simulink model "disturbed_subsystem_old"  (Simulink 9.0)
settings: Solver=ode5  StartTime=0.0  StopTime=30  RelTol=1e-3  AbsTol=1e-6
model workspace: external: MATLAB File workspace.m (data not in the file)
values from neighbouring files (symbols this model uses):
  DOWN_TABLE = [0 5 20 35 ... (first row only)    [workspace.m]
  DOWN_TH_BP = [0; 5; 40; 50; 90; 100]    [workspace.m]
  EMAP = [-40 -44 -49 -53 -57 -61 -65 -70 -74 -78 -82 ... (first row only)    [workspace.m]
  Iei = 0.021991488283555904    (= 0.0219914882836)    [workspace.m]
  NE_VEC = [799.99999999999989 1200 1599.9999999999998 1999.9999999999998            2400 2800.0000000000005 3199.9999999999995 3599.9999999999995            3999.9999999999995 4400 4800]    [workspace.m]
  TH_VEC = [0; 20; 30; 40; 50; 60; 70; 80; 90; 100]    [workspace.m]
  UP_TABLE = [12 30 50 1.0E+6 ... (first row only)    [workspace.m]
  UP_TH_BP = [0; 25; 35; 50; 90; 100]    [workspace.m]
undefined symbols (not defined in the file): CONVERTER_DATA, VEHICLE_DATA
Description:
  | Modeling an Automatic Transmission Controller
  | 
  | In this example, Simulink(R) is used to model an automotive drivetrain. Stateflow(R)
  | enhances the Simulink model with its representation of the transmission
  | control logic. Simulink provides a powerful environment for the modeling and
  | simulation of dynamic systems and processes. In many systems, though,
  | supervisory functions like changing modes or invoking new gain schedules must
  | respond to events that may occur and conditions that develop over time. As a
  | result, the environment requires a language capable of managing these multiple
  | modes and developing conditions. In the following example, Stateflow
  | demonstrates its strength in this capacity by performing the function of gear
  | selection in an automatic transmission. This function is combined with the
  | drivetrain dynamics in a natural and intuitive manner by incorporating a
  | Stateflow block in the Simulink block diagram.
settings Model: SuppressorTable=22 serialization::archive 11 0 6 0 0 0 1 0  DataTypeOverride=Double  MinMaxOverflowLogging=ForceOff  FPTRunName=Active  Creator=The MathWorks, Inc.  LastModifiedBy=luigi  ExtModeTrigMode=oneshot  ExtModeArmWhenConnect=off  ExtModeAutoUpdateStatusClock=off
settings DataIOCC: SaveFormat=StructureWithTime  SaveOutput=off  SaveTime=off  SignalLoggingName=sldemo_autotrans_output
settings OptimizationCC: BlockReduction=off  ExpressionDepthLimit=2147483647  InitFltsAndDblsToZero=on
settings DebuggingCC: SignalInfNanChecking=error  SaveWithParameterizedLinksMsg=none  UnderspecifiedInitializationDetection=Simplified  MergeDetectMultiDrivingBlocksExec=error  CheckExecutionContextPreStartOutputMsg=on  CheckExecutionContextRuntimeOutputMsg=on  MultiTaskCondExecSysMsg=none  SigSpecEnsureSampleTimeMsg=none  IntegerOverflowMsg=none  FcnCallInpInsideContextMsg=warning  SignalLabelMismatchMsg=error  UnconnectedInputMsg=error  UnconnectedOutputMsg=error  UnconnectedLineMsg=error  UniqueDataStoreMsg=error  BusObjectLabelMismatch=error  RootOutportRequireBusObject=error  StateNameClashWarn=warning  StrictBusMsg=ErrorOnBusTreatedAsVector  NonBusSignalsTreatedAsBus=error  IntegerSaturationMsg=none
settings HardwareCC: ProdIntDivRoundTo=Floor
settings SFSimCC: SFSimEcho=off  SimParseCustomCode=off
settings GRTTargetCC: TargetFcnLib=ansi_tfl_tmw.mat  GeneratePreprocessorConditionals=Disable all  CombineOutputUpdateFcns=off  GRTInterface=on
settings ConfigComp: CovMetricSettings=dcmtr  CovHTMLOptions=-aTS=1 -bRG=1 -bTC=1 -hTR=0 -nFC=0 -scm=1 -bcm=1 -xEv=0  CovHtmlReporting=off

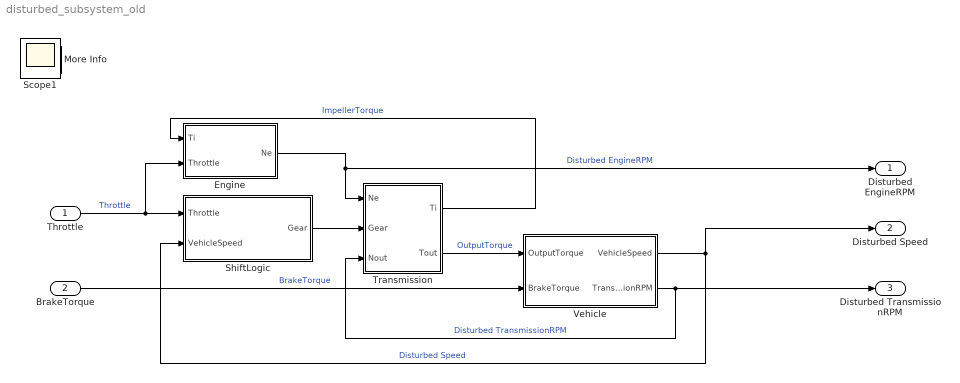
== system disturbed_subsystem_old ==
  Throttle : Inport
  BrakeTorque : Inport  Port=2
  Engine : Subsystem
  More Info : Subsystem
      settings: OpenFcn=showdemo(bdroot(gcb))
      mask Display: disp('?')
  ShiftLogic : Stateflow chart  TreatAsAtomicUnit=on
  Transmission : Subsystem
  Vehicle : Subsystem  mask(vehicle model){Rfd=VEHICLE_DATA(1), rload0=VEHICLE_DATA(2), rload2=VEHICLE_DATA(3), Rw=VEHICLE_DATA(4), Iv=VEHICLE_DATA(5), N20=VEHICLE_DATA(6)/VEHICLE_DATA(4)*VEHICLE_DATA(1)}
      mask prompts: Rfd "final drive ratio"; rload0 "drag friction at wheels"; rload2 "aerodynamic drag"; Rw "wheel radius"; Iv "vehicle inertia"; N20 "initial transmission output speed"
      mask help: vehicle dynamics: torque input from trans., outputs are input speed (transmission output) and vehicle speed
      mask Display: image([matlabroot,'/toolbox/simulink/simdemos/automotive/html/NSX_3Colors.jpg'])
  Disturbed EngineRPM : Outport
  Disturbed Speed : Outport  Port=2
  Disturbed TransmissionRPM : Outport  Port=3
  Scope1 : Scope
  wires:
  Transmission/1(Ti) -> Engine/1(Ti)  "ImpellerTorque"
  Engine/1(Ne) -> Disturbed EngineRPM/1, Transmission/1(Ne)  "Disturbed EngineRPM"
  Transmission/2(Tout) -> Vehicle/1(OutputTorque)  "OutputTorque"
  Vehicle/2(TransmissionRPM) -> Transmission/3(Nout), Disturbed TransmissionRPM/1  "Disturbed TransmissionRPM"
  ShiftLogic/1(Gear) -> Transmission/2(Gear)
  Vehicle/1(VehicleSpeed) -> Disturbed Speed/1, ShiftLogic/2(VehicleSpeed)  "Disturbed Speed"
  Throttle/1 -> Engine/2(Throttle), ShiftLogic/1(Throttle)  "Throttle"
  BrakeTorque/1 -> Vehicle/2(BrakeTorque)  "BrakeTorque"

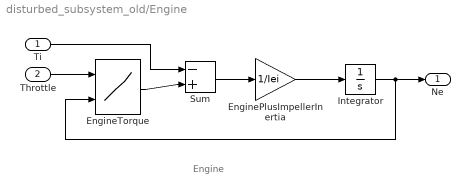
== system disturbed_subsystem_old/Engine ==
  note: Engine
  Ti : Inport  Unit=ft*lbf@torque
  Throttle : Inport  Port=2  Unit=%
  EnginePlusImpellerInertia : Gain  Gain=1/Iei  SaturateOnIntegerOverflow=on  OutDataTypeStr=Inherit: Same as input  ParamDataTypeStr=Inherit: Same as input
  EngineTorque : Lookup_n-D  BreakpointsForDimension1=TH_VEC  BreakpointsForDimension2=NE_VEC  Table=EMAP  InputSameDT=on
  Integrator : Integrator  InitialCondition=1000  LimitOutput=on  UpperSaturationLimit=6000  LowerSaturationLimit=600  ZeroCross=off
  Sum : Sum  Inputs=-+  SaturateOnIntegerOverflow=on  InputSameDT=on  OutDataTypeStr=Inherit: Same as first input
  Ne : Outport  Unit=rpm
  wires:
  Ti/1 -> Sum/1
  Throttle/1 -> EngineTorque/1
  Integrator/1 -> EngineTorque/2, Ne/1
  Sum/1 -> EnginePlusImpellerInertia/1
  EnginePlusImpellerInertia/1 -> Integrator/1
  EngineTorque/1 -> Sum/2

== system disturbed_subsystem_old/More Info ==

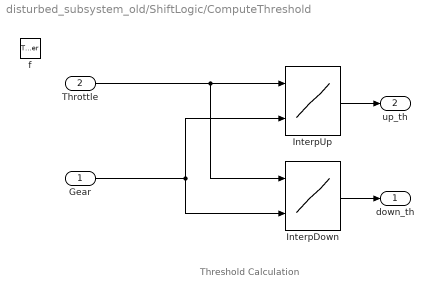
== system disturbed_subsystem_old/ShiftLogic/ComputeThreshold ==
  note: Threshold Calculation
  Gear : Inport
  Throttle : Inport  Port=2
  f : TriggerPort  TriggerType=function-call  VariantControl=(inherit)
      settings: CopyFcn=Stateflow.SLINSF.SimulinkMan.removeBlockPreDeleteFcn  PreDeleteFcn=Stateflow.SLINSF.SimulinkMan.unsafePredeleteFcn
  InterpDown : Lookup_n-D  BreakpointsForDimension1=DOWN_TH_BP  BreakpointsForDimension2=[1:4]  Table=DOWN_TABLE  OutDataTypeStr=double  LockScale=on
  InterpUp : Lookup_n-D  BreakpointsForDimension1=UP_TH_BP  BreakpointsForDimension2=[1:4]  Table=UP_TABLE  OutDataTypeStr=double  LockScale=on
  down_th : Outport  InitialOutput=0
  up_th : Outport  Port=2  InitialOutput=0
  wires:
  InterpUp/1 -> up_th/1
  InterpDown/1 -> down_th/1
  Throttle/1 -> InterpDown/1, InterpUp/1
  Gear/1 -> InterpDown/2, InterpUp/2

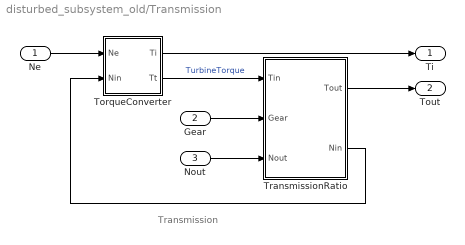
== system disturbed_subsystem_old/Transmission ==
  note: Transmission
  Ne : Inport  Unit=rpm
  Gear : Inport  Port=2  Unit=1
  Nout : Inport  Port=3  Unit=rpm
  TorqueConverter : Subsystem  mask(torque converter){speedratio=CONVERTER_DATA(:,1), Kfactor=CONVERTER_DATA(:,2), Torkratio=CONVERTER_DATA(:,3)}
      mask prompts: speedratio "speed ratio"; Kfactor "K factor"; Torkratio "torque ratio"
      mask help: torque converter
      mask Help: Torque converter input and output torques are computed as a function of the input and output speeds
      mask Display: plot([cos([90:10:450]*pi/180),.63*cos([90:10:450]*pi/180),.63*cos([90:10:240]*pi/180),cos([240:10:300]*pi/180),.63*cos([300]*pi/180)],[sin([90:10:450]*pi/180),.63*sin([90:10:450]*pi/180)+.1,.63*sin([90:10:240]*pi/180)+.1,sin([240:10:300]*pi/180),.63*sin([300]*pi/180)+.1])
  TransmissionRatio : Subsystem
  Ti : Outport  Unit=ft*lbf@torque
  Tout : Outport  Port=2  Unit=ft*lbf@torque
  wires:
  TransmissionRatio/1(Tout) -> Tout/1
  TorqueConverter/1(Ti) -> Ti/1
  Nout/1 -> TransmissionRatio/3(Nout)
  Gear/1 -> TransmissionRatio/2(Gear)
  Ne/1 -> TorqueConverter/1(Ne)
  TransmissionRatio/2(Nin) -> TorqueConverter/2(Nin)
  TorqueConverter/2(Tt) -> TransmissionRatio/1(Tin)  "TurbineTorque"

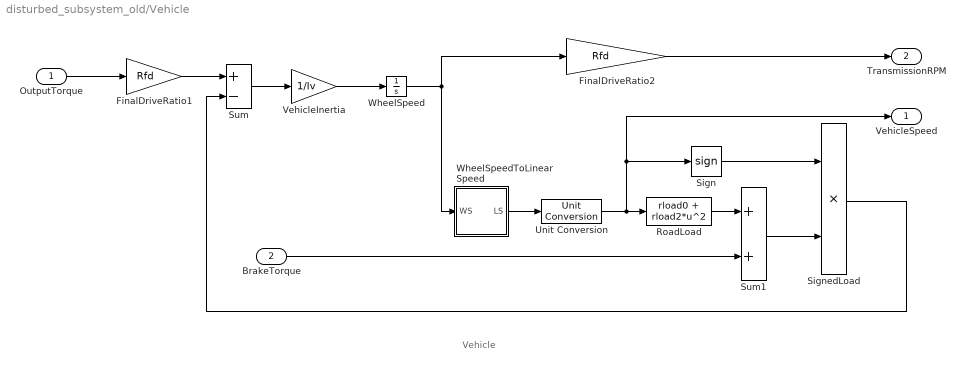
== system disturbed_subsystem_old/Vehicle ==
  note: Vehicle
  OutputTorque : Inport  Unit=ft*lbf@torque
  BrakeTorque : Inport  Port=2  Unit=ft*lbf@torque
  FinalDriveRatio1 : Gain  Gain=Rfd  SaturateOnIntegerOverflow=on  OutDataTypeStr=Inherit: Same as input  ParamDataTypeStr=Inherit: Same as input
  FinalDriveRatio2 : Gain  Gain=Rfd  SaturateOnIntegerOverflow=on  OutDataTypeStr=Inherit: Same as input  ParamDataTypeStr=Inherit: Same as input
  RoadLoad : Fcn  Expr=rload0 + rload2*u^2
  Sign : Signum
  SignedLoad : Product  SaturateOnIntegerOverflow=on  InputSameDT=on  OutDataTypeStr=Inherit: Same as first input
  Sum : Sum  Inputs=+-  SaturateOnIntegerOverflow=on  InputSameDT=on  OutDataTypeStr=Inherit: Same as first input
  Sum1 : Sum  SaturateOnIntegerOverflow=on  InputSameDT=on  OutDataTypeStr=Inherit: Same as first input
  Unit Conversion : UnitConversion
  VehicleInertia : Gain  Gain=1/Iv  SaturateOnIntegerOverflow=on  OutDataTypeStr=Inherit: Same as input  ParamDataTypeStr=Inherit: Same as input
  WheelSpeed : Integrator  InitialCondition=N20/Rfd  ZeroCross=off
  WheelSpeedToLinearSpeed : Subsystem
  VehicleSpeed : Outport  Unit=mph
  TransmissionRPM : Outport  Port=2  Unit=rpm
  wires:
  FinalDriveRatio2/1 -> TransmissionRPM/1
  BrakeTorque/1 -> Sum1/2
  Sum1/1 -> SignedLoad/2
  RoadLoad/1 -> Sum1/1
  Sign/1 -> SignedLoad/1
  SignedLoad/1 -> Sum/2
  OutputTorque/1 -> FinalDriveRatio1/1
  VehicleInertia/1 -> WheelSpeed/1
  Sum/1 -> VehicleInertia/1
  Unit Conversion/1 -> VehicleSpeed/1, Sign/1, RoadLoad/1
  WheelSpeed/1 -> WheelSpeedToLinearSpeed/1(WS), FinalDriveRatio2/1
  FinalDriveRatio1/1 -> Sum/1
  WheelSpeedToLinearSpeed/1(LS) -> Unit Conversion/1

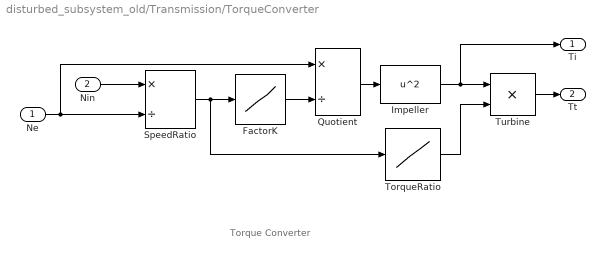
== system disturbed_subsystem_old/Transmission/TorqueConverter ==
  note: Torque Converter
  Ne : Inport
  Nin : Inport  Port=2
  FactorK : Lookup_n-D  NumberOfTableDimensions=1  BreakpointsForDimension1=speedratio  Table=Kfactor  SaturateOnIntegerOverflow=on  InputSameDT=on
  Impeller : Fcn  Expr=u^2
  Quotient : Product  Inputs=*/  SaturateOnIntegerOverflow=on  InputSameDT=on  OutDataTypeStr=Inherit: Same as first input
  SpeedRatio : Product  Inputs=*/  SaturateOnIntegerOverflow=on  InputSameDT=on  OutDataTypeStr=Inherit: Same as first input
  TorqueRatio : Lookup_n-D  NumberOfTableDimensions=1  BreakpointsForDimension1=speedratio  Table=Torkratio  SaturateOnIntegerOverflow=on  InputSameDT=on
  Turbine : Product  SaturateOnIntegerOverflow=on  InputSameDT=on  OutDataTypeStr=Inherit: Same as first input
  Ti : Outport
  Tt : Outport  Port=2
  wires:
  TorqueRatio/1 -> Turbine/2
  Quotient/1 -> Impeller/1
  FactorK/1 -> Quotient/2
  SpeedRatio/1 -> TorqueRatio/1, FactorK/1
  Impeller/1 -> Turbine/1, Ti/1
  Turbine/1 -> Tt/1
  Ne/1 -> SpeedRatio/2, Quotient/1
  Nin/1 -> SpeedRatio/1

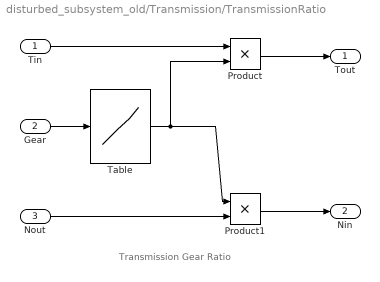
== system disturbed_subsystem_old/Transmission/TransmissionRatio ==
  note: Transmission Gear Ratio
  Tin : Inport  Unit=ft*lbf@torque
  Gear : Inport  Port=2  Unit=1
  Nout : Inport  Port=3  Unit=rpm
  Product : Product  SaturateOnIntegerOverflow=on  InputSameDT=on  OutDataTypeStr=Inherit: Same as first input
  Product1 : Product  SaturateOnIntegerOverflow=on  InputSameDT=on  OutDataTypeStr=Inherit: Same as first input
  Table : Lookup_n-D  NumberOfTableDimensions=1  BreakpointsForDimension1=[1 2 3 4]  Table=[2.393 1.450 1.000 0.677]  OutDataTypeStr=double  SaturateOnIntegerOverflow=on  InputSameDT=on  LockScale=on
  Tout : Outport  Unit=ft*lbf@torque
  Nin : Outport  Port=2  Unit=rpm
  wires:
  Table/1 -> Product1/1, Product/2
  Nout/1 -> Product1/2
  Product1/1 -> Nin/1
  Product/1 -> Tout/1
  Tin/1 -> Product/1
  Gear/1 -> Table/1

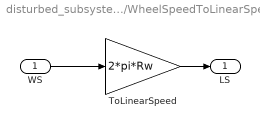
== system disturbed_subsystem_old/Vehicle/WheelSpeedToLinearSpeed ==
  WS : Inport  Unit=rpm
  ToLinearSpeed : Gain  Gain=2*pi*Rw  SaturateOnIntegerOverflow=on  OutDataTypeStr=Inherit: Same as input  ParamDataTypeStr=Inherit: Same as input
  LS : Outport  Unit=ft/min
  wires:
  ToLinearSpeed/1 -> LS/1
  WS/1 -> ToLinearSpeed/1

== stateflow chart ShiftLogic ==
  settings: updateMethod=DISCRETE  sampleTime=0.04
  state gear_state [parallel]
    settings: executionOrder=1
    state first
      entry:
      Gear = 1;
    state second
      entry:
      Gear = 2;
    state third
      entry:
      Gear = 3;
    state fourth
      entry:
      Gear = 4;
    (default) -> first
    second -> third [order 1] : UP
    first -> second : UP
    third -> fourth [order 1] : UP
    third -> second [order 2] : DOWN
    second -> first [order 2] : DOWN
    fourth -> third : DOWN
  state selection_state [parallel]
    during:
    [down_th, up_th] = ComputeThreshold(Gear,Throttle);
    settings: executionOrder=2
    state steady_state
    state upshifting
    state downshifting
    (default) -> steady_state
    steady_state -> upshifting [order 1] : [VehicleSpeed > up_th]
    steady_state -> downshifting [order 2] : [VehicleSpeed < down_th]
    downshifting -> steady_state [order 2] : [VehicleSpeed > down_th]
    downshifting -> steady_state [order 1] : after(TWAIT,tick)
        | [VehicleSpeed <= down_th]
        | {gear_state.DOWN}
    upshifting -> steady_state [order 1] : after(TWAIT,tick)
        | [VehicleSpeed >= up_th]
        | {gear_state.UP}
    upshifting -> steady_state [order 2] : [VehicleSpeed < up_th]
  state [down_th,up_th] = ComputeThreshold(Gear,Throttle) [function]
  data: Gear function_input double; Throttle function_input double; down_th function_output double; up_th function_output double; Throttle input double; VehicleSpeed input double; Gear output fixdt(0,8,5) [1..4]; TWAIT parameter fixdt(0,8,6); down_th local double; up_th local double
  events: DOWN local EITHER_EDGE_EVENT; UP local EITHER_EDGE_EVENT
